simulink model "zumo_PID_controller_line_value"  (R2014b)
settings: Solver=ode3  SolverMode=SingleTasking  StartTime=0.0  StopTime=20  FixedStep=0.01  RelTol=1e-3
PreLoadFcn:
  | evalin('base','sim=1;');
InitFcn:
  | mapdata = processmap('mapTrackA.mat');
model workspace (MAT data in the model file):
  axleLength = Simulink.Parameter
  axleLength.Value = 9.8
  axleLength.Description = 'Distance between tire contact points
    | of the two wheels/treads
    | in units of centimeters.'
  axleLength.DataType = 'auto'
  commandPercmPerSecond = Simulink.Parameter
  commandPercmPerSecond.Value = 3.9547
  commandPercmPerSecond.Description = 'Convert units of ''command'' 
    | to units of ''cm/s''.
    | 
    | ''command'' is a value in the range [-256, 255].'
  commandPercmPerSecond.DataType = 'auto'
  symmetrizeMotors = Simulink.Parameter
  symmetrizeMotors.Value = 1
  symmetrizeMotors.Description = 'Scale one of the motor commands down 
    | (not up) to balance the motors. 
    | Once balanced, a value of x sent to either
    | motor will produce the same rate of rotation
    | in both motors.'
  symmetrizeMotors.DataType = 'auto'
  sampleTime = Simulink.Parameter
  sampleTime.Value = 0.01
  sampleTime.Description = 'Sample time (in seconds) of the trajectory simulator.'
  sampleTime.DataType = 'auto'
  commandThreshold = Simulink.Parameter
  commandThreshold.Value = 31.875
  commandThreshold.DataType = 'auto'
  lineThreshold = Simulink.Parameter
  lineThreshold.Value = 500
  lineThreshold.DataType = 'auto'
  velocity = Simulink.Parameter
  velocity.Value = 10
  velocity.Description = 'cm / s'
  velocity.DataType = 'auto'
  waveLength = Simulink.Parameter
  waveLength.Value = 8.6
  waveLength.Description = 'Units of cm.
    | 
    | The following condition must be satisfied: 
    | waveLength > 2*pi * velocity / sqrt(0.5 / sampleTime)
    | 
    | For reference,
    | robotLength = 8.6 cm
    | '
  waveLength.DataType = 'auto'
libraries: ZumoBotLib x2, simulink x1, arduinolib x1
settings Model: ExtModeTrigDuration=2  Creator=pkasseba  LastModifiedBy=sandip
settings OptimizationCC: OptimizeModelRefInitCode=on  LifeSpan=1
settings DebuggingCC: UnderspecifiedInitializationDetection=Classic  MergeDetectMultiDrivingBlocksExec=none  SolverPrmCheckMsg=none  StateNameClashWarn=warning
settings HardwareCC: ProdBitPerInt=16  ProdBitPerPointer=8  ProdIntDivRoundTo=Zero  ProdEndianess=LittleEndian  ProdWordSize=8  ProdHWDeviceType=Atmel->AVR
settings SFSimCC: SimParseCustomCode=off
settings RTWCC: SystemTargetFile=realtime.tlc  GenerateMakefile=off  TemplateMakefile=realtime.tmf  Description=Run on Target Hardware  RTWVerbose=off  ProcessScript=realtime_make_rtw_hook
settings STFCustomTargetCC: TargetLibSuffix=.a  GenerateSampleERTMain=on  ERTCustomFileBanners=on  SupportNonInlinedSFcns=off  SupportVariableSizeSignals=on  MATLABClassNameForMDSCustomization=Simulink.SoftwareTarget.ERTCustomization  GRTInterface=off  SystemTargetFile=realtime.tlc
settings ERTTargetCC: GenerateSampleERTMain=on  ParMdlRefBuildCompliant=off  CompOptLevelCompliant=off  ConcurrentExecutionCompliant=off  CombineOutputUpdateFcns=off  ERTFirstTimeCompliant=off  SupportContinuousTime=on  SupportVariableSizeSignals=on  ModelStepFunctionPrototypeControlCompliant=off  CPPClassGenCompliant=off  ExtModeTransport=3  ExtModeMexFile=ext_serial_win32_comm  ExtModeMexArgs=0 1 9600  InlinedParameterPlacement=NonHierarchical  ERTSrcFileBannerTemplate=realtime_code_template.cgt  ERTHdrFileBannerTemplate=realtime_code_template.cgt  ERTDataSrcFileTemplate=realtime_code_template.cgt  ERTDataHdrFileTemplate=realtime_code_template.cgt  ERTCustomFileTemplate=realtime_file_process.tlc

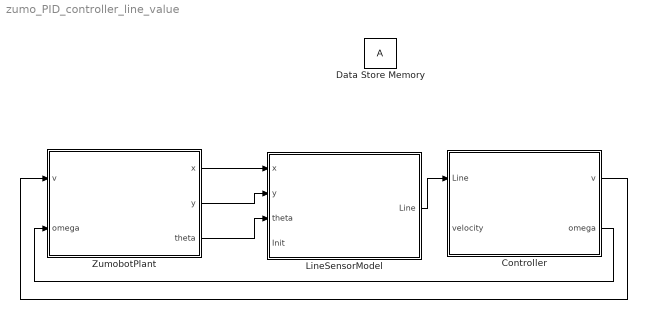
== system zumo_PID_controller_line_value ==
  Controller : Subsystem
  Data Store Memory : DataStoreMemory  Priority=2  ReadBeforeWriteMsg=warning  WriteAfterWriteMsg=warning  WriteAfterReadMsg=warning
  LineSensorModel : Subsystem  Variant=on
  ZumobotPlant : Subsystem  Variant=on
  wires:
  Controller/1(v) -> ZumobotPlant/1(v)
  ZumobotPlant/2(y) -> LineSensorModel/2(y)
  LineSensorModel/1(Line) -> Controller/1(Line)
  Controller/2(omega) -> ZumobotPlant/2(omega)
  ZumobotPlant/3(theta) -> LineSensorModel/3(theta)
  ZumobotPlant/1(x) -> LineSensorModel/1(x)

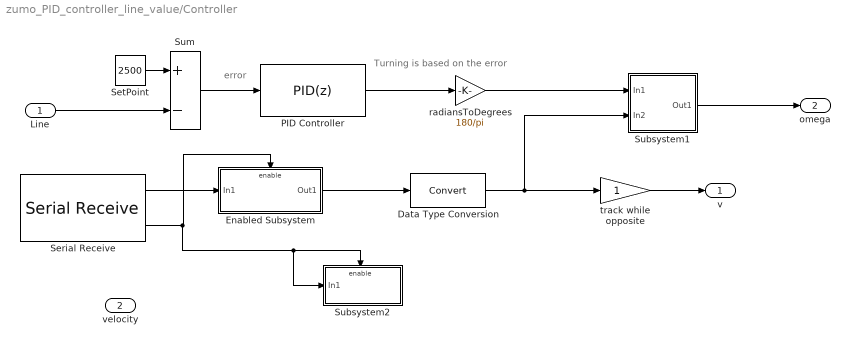
== system zumo_PID_controller_line_value/Controller ==
  note: Turning is based on the error
  note: error
  Line : Inport
  velocity : Inport  Port=2
  Data Type Conversion : DataTypeConversion
  Enabled Subsystem : Subsystem  TreatAsAtomicUnit=on
  PID Controller : simulink/Continuous/PID Controller  Controller=PID  TimeDomain=Discrete-time  SampleTime=-1  IntegratorMethod=Forward Euler  FilterMethod=Forward Euler  Form=Parallel  P=0.01  I=0.01  D=0.005  N=1  InitialConditionSource=internal  InitialConditionForIntegrator=0  InitialConditionForFilter=0  ExternalReset=none  LimitOutput=off  UpperSaturationLimit=5  LowerSaturationLimit=-5  LinearizeAsGain=on  AntiWindupMode=none  Kb=1  TrackingMode=off  Kt=1  PParamMin=[]  PParamMax=[]  IParamMin=[]  IParamMax=[]  DParamMin=[]  DParamMax=[]  NParamMin=[]  NParamMax=[]  KbParamMin=[]  KbParamMax=[]  KtParamMin=[]  KtParamMax=[]  POutMin=[]  POutMax=[]  IOutMin=[]  IOutMax=[]  DOutMin=[]  DOutMax=[]  NOutMin=[]  NOutMax=[]  KbOutMin=[]  KbOutMax=[]  KtOutMin=[]  KtOutMax=[]  IntegratorOutMin=[]  IntegratorOutMax=[]  FilterOutMin=[]  FilterOutMax=[]  SumOutMin=[]  SumOutMax=[]  SumI1OutMin=[]  SumI1OutMax=[]  SumI2OutMin=[]  SumI2OutMax=[]  SumI3OutMin=[]  SumI3OutMax=[]  SumDOutMin=[]  SumDOutMax=[]  SaturationOutMin=[]  SaturationOutMax=[]  IntegratorContinuousStateAttributes=''  IntegratorStateMustResolveToSignalObject=off  IntegratorRTWStateStorageClass=Auto  FilterContinuousStateAttributes=''  FilterStateMustResolveToSignalObject=off  FilterRTWStateStorageClass=Auto  DifferentiatorICPrevScaledInput=0  DifferentiatorOutMin=[]  DifferentiatorOutMax=[]  UseFilter=on
  Serial Receive : arduinolib/Serial Receive  portNumber=0  showOutStatus=on  sampleTime=0.01  blockPlatform=arduino
  SetPoint : Constant  Value=2500
  Subsystem1 : Subsystem
  Subsystem2 : Subsystem  Priority=0
  Sum : Sum  Inputs=+-
  radiansToDegrees : Gain  Gain=180/pi
  track while opposite : Gain
  v : Outport
  omega : Outport  Port=2
  wires:
  SetPoint/1 -> Sum/1
  Sum/1 -> PID Controller/1
  PID Controller/1 -> radiansToDegrees/1
  Line/1 -> Sum/2
  Data Type Conversion/1 -> Subsystem1/2(In2), track while opposite/1
  track while opposite/1 -> v/1
  radiansToDegrees/1 -> Subsystem1/1(In1)
  Subsystem1/1(Out1) -> omega/1
  Serial Receive/1 -> Enabled Subsystem/1(In1)
  Enabled Subsystem/1(Out1) -> Data Type Conversion/1
  Serial Receive/2 -> Subsystem2/1(In1), Subsystem2/Enable, Enabled Subsystem/Enable

== system zumo_PID_controller_line_value/LineSensorModel ==
  note: 1) Only subsystems can be added as variant choices at this level
      | 2) Blocks cannot be connected at this level as connectivity is
      | automatically determined at simulation, based on the active variant
  x : Inport
  y : Inport  Port=2
  theta : Inport  Port=3
  Init : Inport  Port=4
  Simulation : Subsystem  VariantControl=sim==1
  Target : Subsystem  VariantControl=sim==0
  Line : Outport

== system zumo_PID_controller_line_value/ZumobotPlant ==
  note: 1) Only subsystems can be added as variant choices at this level
      | 2) Blocks cannot be connected at this level as connectivity is
      | automatically determined at simulation, based on the active variant
  v : Inport
  omega : Inport  Port=2
  Simulation : Subsystem  VariantControl=sim==1
  Target : Subsystem  VariantControl=sim==0
  x : Outport
  y : Outport  Port=2
  theta : Outport  Port=3

== system zumo_PID_controller_line_value/Controller/Enabled Subsystem ==
  In1 : Inport
  Enable : EnablePort
  Out1 : Outport  InitialOutput=0
  wires:
  In1/1 -> Out1/1

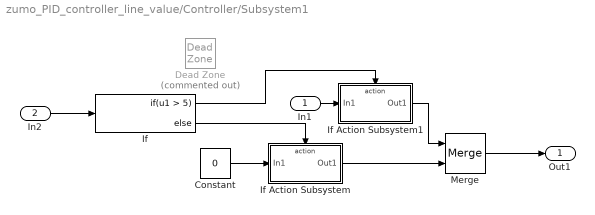
== system zumo_PID_controller_line_value/Controller/Subsystem1 ==
  In1 : Inport
  In2 : Inport  Port=2
  Constant : Constant  Value=0
  Dead Zone : DeadZone  Commented=on  LowerValue=-5  UpperValue=5  SaturateOnIntegerOverflow=on
  If : If  IfExpression=u1 > 5
  If Action Subsystem : Subsystem  TreatAsAtomicUnit=on
  If Action Subsystem1 : Subsystem  TreatAsAtomicUnit=on
  Merge : Merge
  Out1 : Outport
  wires:
  If/2 -> If Action Subsystem/Action
  Merge/1 -> Out1/1
  In2/1 -> If/1
  If Action Subsystem/1(Out1) -> Merge/2
  If Action Subsystem1/1(Out1) -> Merge/1
  In1/1 -> If Action Subsystem1/1(In1)
  Constant/1 -> If Action Subsystem/1(In1)
  If/1 -> If Action Subsystem1/Action

== system zumo_PID_controller_line_value/Controller/Subsystem2 ==
  In1 : Inport
  Enable : EnablePort
  Data Store Write : DataStoreWrite  DataStoreElements=A
  wires:
  In1/1 -> Data Store Write/1

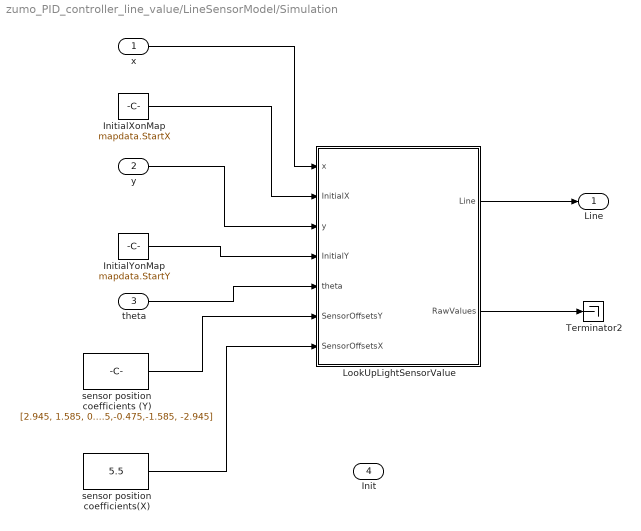
== system zumo_PID_controller_line_value/LineSensorModel/Simulation ==
  x : Inport
  y : Inport  Port=2
  theta : Inport  Port=3
  Init : Inport  Port=4
  InitialXonMap : Constant  Value=mapdata.StartX
  InitialYonMap : Constant  Value=mapdata.StartY
  LookUpLightSensorValue : Subsystem
  Terminator2 : Terminator
  sensor position coefficients (Y) : Constant  Value=[2.945, 1.585, 0.475,-0.475,-1.585, -2.945]
  sensor position coefficients(X) : Constant  Value=5.5
  Line : Outport
  wires:
  InitialYonMap/1 -> LookUpLightSensorValue/4(InitialY)
  theta/1 -> LookUpLightSensorValue/5(theta)
  sensor position coefficients (Y)/1 -> LookUpLightSensorValue/6(SensorOffsetsY)
  y/1 -> LookUpLightSensorValue/3(y)
  InitialXonMap/1 -> LookUpLightSensorValue/2(InitialX)
  x/1 -> LookUpLightSensorValue/1(x)
  sensor position coefficients(X)/1 -> LookUpLightSensorValue/7(SensorOffsetsX)
  LookUpLightSensorValue/1(Line) -> Line/1
  LookUpLightSensorValue/2(RawValues) -> Terminator2/1

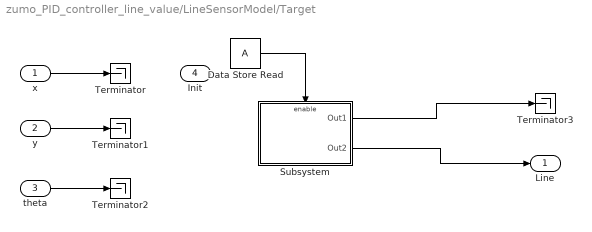
== system zumo_PID_controller_line_value/LineSensorModel/Target ==
  x : Inport
  y : Inport  Port=2
  theta : Inport  Port=3
  Init : Inport  Port=4
  Data Store Read : DataStoreRead
  Subsystem : Subsystem
  Terminator{,1..3} (4 alike) : Terminator
  Line : Outport
  wires:
  x/1 -> Terminator/1
  y/1 -> Terminator1/1
  theta/1 -> Terminator2/1
  Subsystem/1(Out1) -> Terminator3/1
  Subsystem/2(Out2) -> Line/1
  Data Store Read/1 -> Subsystem/Enable

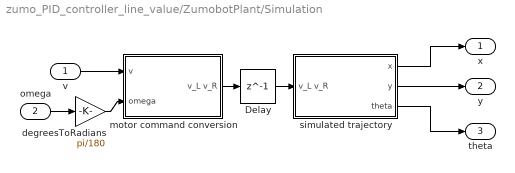
== system zumo_PID_controller_line_value/ZumobotPlant/Simulation ==
  v : Inport
  omega : Inport  Port=2
  Delay : Delay  DelayLength=1  InitialCondition=0
  degreesToRadians : Gain  Gain=pi/180
  motor command conversion : Subsystem
  simulated trajectory : Subsystem
  x : Outport
  y : Outport  Port=2
  theta : Outport  Port=3
  wires:
  v/1 -> motor command conversion/1(v)
  simulated trajectory/1(x) -> x/1
  simulated trajectory/2(y) -> y/1
  omega/1 -> degreesToRadians/1
  simulated trajectory/3(theta) -> theta/1
  degreesToRadians/1 -> motor command conversion/2(omega)
  motor command conversion/1(v_L v_R) -> Delay/1
  Delay/1 -> simulated trajectory/1(v_L v_R)

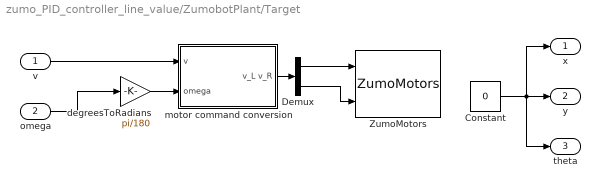
== system zumo_PID_controller_line_value/ZumobotPlant/Target ==
  v : Inport
  omega : Inport  Port=2
  Constant : Constant  Value=0
  Demux : Demux  Outputs=2
  ZumoMotors : ZumoBotLib/ZumoMotors  flipLeft=off  flipRight=off
  degreesToRadians : Gain  Gain=pi/180
  motor command conversion : Subsystem
  x : Outport
  y : Outport  Port=2
  theta : Outport  Port=3
  wires:
  motor command conversion/1(v_L v_R) -> Demux/1
  Demux/1 -> ZumoMotors/1
  Demux/2 -> ZumoMotors/2
  v/1 -> motor command conversion/1(v)
  omega/1 -> degreesToRadians/1
  Constant/1 -> theta/1, x/1, y/1
  degreesToRadians/1 -> motor command conversion/2(omega)

== system zumo_PID_controller_line_value/Controller/Subsystem1/If Action Subsystem ==
  In1 : Inport
  Action Port : ActionPort  ActionType=else
  Out1 : Outport
  wires:
  In1/1 -> Out1/1

== system zumo_PID_controller_line_value/Controller/Subsystem1/If Action Subsystem1 ==
  In1 : Inport
  Action Port : ActionPort  ActionType=then
  Out1 : Outport
  wires:
  In1/1 -> Out1/1

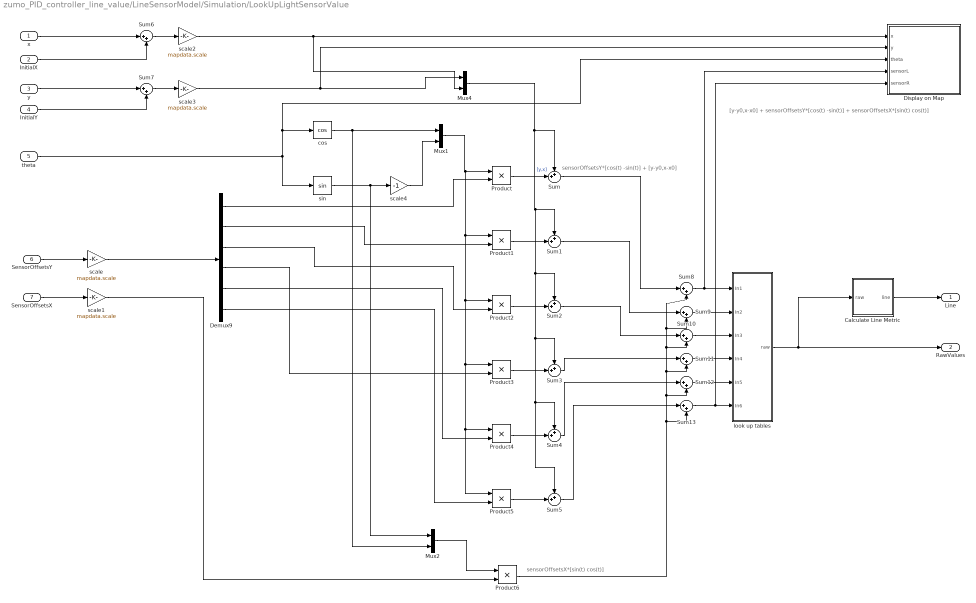
== system zumo_PID_controller_line_value/LineSensorModel/Simulation/LookUpLightSensorValue ==
  note: [y-y0,x-x0] + sensorOffsetsY*[cos(t) -sin(t)] + sensorOffsetsX*[sin(t) cos(t)]
  note: sensorOffsetsY*[cos(t) -sin(t)] + [y-y0,x-x0]
  note: sensorOffsetsX*[sin(t) cos(t)]
  x : Inport
  InitialX : Inport  Port=2
  y : Inport  Port=3
  InitialY : Inport  Port=4
  theta : Inport  Port=5
  SensorOffsetsY : Inport  Port=6
  SensorOffsetsX : Inport  Port=7
  Calculate Line Metric : Subsystem
  Demux9 : Demux  Outputs=6
  Display on Map : MATLAB Function  TreatAsAtomicUnit=on
  Mux1 : Mux  Inputs=2
  Mux2 : Mux  Inputs=2
  Mux4 : Mux  Inputs=2
  Product{,1..6} (7 alike) : Product
  Sum{,1..5} (6 alike) : Sum  Inputs=++|
  Sum{6..13} (8 alike) : Sum  Inputs=|++
  cos : Trigonometry  Operator=cos
  look up tables : Subsystem
  scale{,1..3} (4 alike) : Gain  Gain=mapdata.scale
  scale4 : Gain  Gain=-1
  sin : Trigonometry
  Line : Outport
  RawValues : Outport  Port=2
  wires:
  SensorOffsetsY/1 -> scale/1
  Mux1/1 -> Product5/1, Product4/1, Product3/1, Product2/1, Product1/1, Product/1
  Product/1 -> Sum/2
  Product1/1 -> Sum1/2
  Product2/1 -> Sum2/2
  Product4/1 -> Sum4/2
  Product3/1 -> Sum3/2
  Product5/1 -> Sum5/2
  Sum/1 -> Sum8/1
  Sum5/1 -> Sum13/1
  scale/1 -> Demux9/1
  Demux9/4 -> Product3/2
  Demux9/5 -> Product4/2
  Demux9/3 -> Product2/2
  Demux9/6 -> Product5/2
  Demux9/2 -> Product1/2
  Demux9/1 -> Product/2
  Mux4/1 -> Sum/1, Sum5/1, Sum4/1, Sum3/1, Sum2/1, Sum1/1  "[y,x]"
  SensorOffsetsX/1 -> scale1/1
  scale1/1 -> Product6/2
  Mux2/1 -> Product6/1
  Product6/1 -> Sum13/2, Sum12/2, Sum11/2, Sum10/2, Sum9/2, Sum8/2
  x/1 -> Sum6/1
  Sum6/1 -> scale2/1
  InitialX/1 -> Sum6/2
  y/1 -> Sum7/1
  Sum7/1 -> scale3/1
  InitialY/1 -> Sum7/2
  scale2/1 -> Mux4/2, Display on Map/1(x)
  scale3/1 -> Mux4/1, Display on Map/2(y)
  Calculate Line Metric/1(line) -> Line/1
  look up tables/1(raw) -> Calculate Line Metric/1(raw), RawValues/1
  Sum1/1 -> Sum9/1
  Sum2/1 -> Sum10/1
  Sum3/1 -> Sum11/1
  Sum4/1 -> Sum12/1
  Sum8/1 -> Display on Map/4(sensorL), look up tables/1(In1)
  Sum9/1 -> look up tables/2(In2)
  Sum10/1 -> look up tables/3(In3)
  Sum11/1 -> look up tables/4(In4)
  Sum12/1 -> look up tables/5(In5)
  Sum13/1 -> Display on Map/5(sensorR), look up tables/6(In6)
  sin/1 -> Mux2/1, scale4/1
  cos/1 -> Mux2/2, Mux1/1
  theta/1 -> Display on Map/3(theta), cos/1, sin/1
  scale4/1 -> Mux1/2

== system zumo_PID_controller_line_value/LineSensorModel/Target/Subsystem ==
  Enable : EnablePort
  ZumoReflectanceSensor : ZumoBotLib/ZumoReflectanceSensor  sampleTime_dd=0.01  emitterPin_dd=255  debug_dd=off
  Out1 : Outport
  Out2 : Outport  Port=2  InitialOutput=2500
  wires:
  ZumoReflectanceSensor/2 -> Out2/1
  ZumoReflectanceSensor/1 -> Out1/1

== system zumo_PID_controller_line_value/ZumobotPlant/Simulation/motor command conversion ==
  note: or in matrix notation,
  note: v_L  = v - omega * axleLength/2
      | v_R = v + omega * axleLength/2
  note: [v_L; v_R] = [1 -axleLength/2; 1 axleLength/2] * [v; omega]
  v : Inport
  omega : Inport  Port=2
  Mux : Mux  Inputs=2
  Saturation [-256 255] : Saturate  UpperLimit=255  LowerLimit=-256
  change parameters : Gain  Gain=[1 -axleLength/2; 1 axleLength/2]  Multiplication=Matrix(K*u)
  change units : Gain  Gain=commandPercmPerSecond
  symmetrize motors : Gain  Gain=[1 symmetrizeMotors]
  v_L v_R : Outport
  wires:
  change parameters/1 -> symmetrize motors/1  "v_L v_R"
  change units/1 -> Saturation [-256 255]/1  "v_L v_R (command)"
  symmetrize motors/1 -> change units/1  "v_L v_R (cm/s)"
  Saturation [-256 255]/1 -> v_L v_R/1
  Mux/1 -> change parameters/1
  omega/1 -> Mux/2
  v/1 -> Mux/1

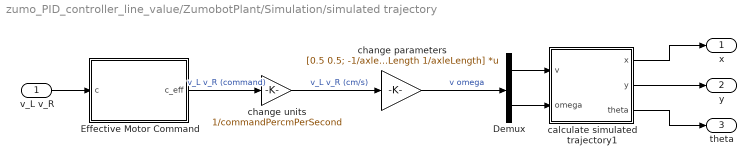
== system zumo_PID_controller_line_value/ZumobotPlant/Simulation/simulated trajectory ==
  v_L v_R : Inport
  Demux : Demux  Outputs=2
  Effective Motor Command : Subsystem
  calculate simulated trajectory1 : Subsystem
  change parameters : Gain  Gain=[0.5 0.5; -1/axleLength 1/axleLength]  Multiplication=Matrix(K*u)
  change units : Gain  Gain=1/commandPercmPerSecond
  x : Outport
  y : Outport  Port=2
  theta : Outport  Port=3
  wires:
  Demux/2 -> calculate simulated trajectory1/2(omega)
  Demux/1 -> calculate simulated trajectory1/1(v)
  v_L v_R/1 -> Effective Motor Command/1(c)
  Effective Motor Command/1(c_eff) -> change units/1  "v_L v_R (command)"
  change units/1 -> change parameters/1  "v_L v_R (cm/s)"
  change parameters/1 -> Demux/1  "v omega"
  calculate simulated trajectory1/2(y) -> y/1
  calculate simulated trajectory1/3(theta) -> theta/1
  calculate simulated trajectory1/1(x) -> x/1

== system zumo_PID_controller_line_value/ZumobotPlant/Target/motor command conversion ==
  note: or in matrix notation,
  note: v_L  = v - omega * axleLength/2
      | v_R = v + omega * axleLength/2
  note: [v_L; v_R] = [1 -axleLength/2; 1 axleLength/2] * [v; omega]
  v : Inport
  omega : Inport  Port=2
  Mux : Mux  Inputs=2
  Saturation [-256 255] : Saturate  UpperLimit=255  LowerLimit=-256
  change parameters : Gain  Gain=[1 -axleLength/2; 1 axleLength/2]  Multiplication=Matrix(K*u)
  change units : Gain  Gain=commandPercmPerSecond
  symmetrize motors : Gain  Gain=[1 symmetrizeMotors]
  v_L v_R : Outport
  wires:
  change parameters/1 -> symmetrize motors/1  "v_L v_R"
  change units/1 -> Saturation [-256 255]/1  "v_L v_R (command)"
  symmetrize motors/1 -> change units/1  "v_L v_R (cm/s)"
  Saturation [-256 255]/1 -> v_L v_R/1
  Mux/1 -> change parameters/1
  omega/1 -> Mux/2
  v/1 -> Mux/1

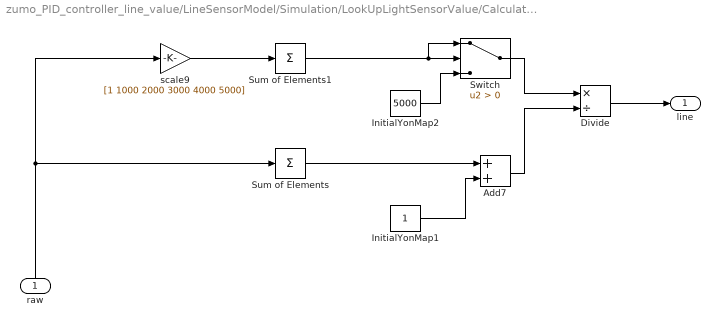
== system zumo_PID_controller_line_value/LineSensorModel/Simulation/LookUpLightSensorValue/Calculate Line Metric ==
  raw : Inport
  Add7 : Sum
  Divide : Product  Inputs=*/
  InitialYonMap1 : Constant
  InitialYonMap2 : Constant  Value=5000
  Sum of Elements : Sum  Inputs=+
  Sum of Elements1 : Sum  Inputs=+
  Switch : Switch  Criteria=u2 > Threshold
  scale9 : Gain  Gain=[1 1000 2000 3000 4000 5000]
  line : Outport
  wires:
  Sum of Elements/1 -> Add7/1
  Divide/1 -> line/1
  InitialYonMap1/1 -> Add7/2
  Add7/1 -> Divide/2
  Sum of Elements1/1 -> Switch/1, Switch/2
  Switch/1 -> Divide/1
  InitialYonMap2/1 -> Switch/3
  scale9/1 -> Sum of Elements1/1
  raw/1 -> scale9/1, Sum of Elements/1

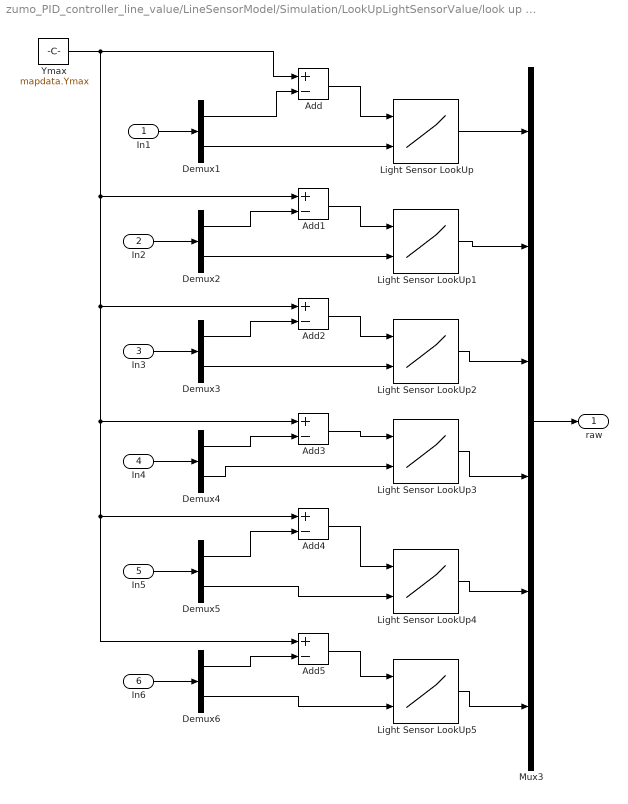
== system zumo_PID_controller_line_value/LineSensorModel/Simulation/LookUpLightSensorValue/look up tables ==
  In1 : Inport
  In2 : Inport  Port=2
  In3 : Inport  Port=3
  In4 : Inport  Port=4
  In5 : Inport  Port=5
  In6 : Inport  Port=6
  Add{,1..5} (6 alike) : Sum  Inputs=+-
  Demux{1..6} (6 alike) : Demux  Outputs=2
  Light Sensor LookUp{,1..5} (6 alike) : Lookup_n-D  BreakpointsForDimension1=mapdata.yBreakPoints  BreakpointsForDimension2=mapdata.xBreakPoints  Table=mapdata.ReflectanceData  InterpMethod=Flat  ExtrapMethod=Clip  UseLastTableValue=on  RndMeth=Round  SaturateOnIntegerOverflow=on  InputSameDT=on
  Mux3 : Mux  Inputs=6
  Ymax : Constant  Value=mapdata.Ymax
  raw : Outport
  wires:
  Demux1/1 -> Add/2
  Demux1/2 -> Light Sensor LookUp/2
  Demux2/2 -> Light Sensor LookUp1/2
  In2/1 -> Demux2/1
  Demux3/2 -> Light Sensor LookUp2/2
  Demux4/2 -> Light Sensor LookUp3/2
  Demux5/2 -> Light Sensor LookUp4/2
  Demux6/2 -> Light Sensor LookUp5/2
  In3/1 -> Demux3/1
  In4/1 -> Demux4/1
  In5/1 -> Demux5/1
  Light Sensor LookUp4/1 -> Mux3/5
  Light Sensor LookUp1/1 -> Mux3/2
  Light Sensor LookUp5/1 -> Mux3/6
  Light Sensor LookUp3/1 -> Mux3/4
  Light Sensor LookUp2/1 -> Mux3/3
  Light Sensor LookUp/1 -> Mux3/1
  Mux3/1 -> raw/1
  Add/1 -> Light Sensor LookUp/1
  Demux2/1 -> Add1/2
  Add1/1 -> Light Sensor LookUp1/1
  Demux3/1 -> Add2/2
  Add2/1 -> Light Sensor LookUp2/1
  Demux4/1 -> Add3/2
  Add3/1 -> Light Sensor LookUp3/1
  Demux5/1 -> Add4/2
  Add4/1 -> Light Sensor LookUp4/1
  Demux6/1 -> Add5/2
  Ymax/1 -> Add5/1, Add4/1, Add3/1, Add2/1, Add1/1, Add/1
  Add5/1 -> Light Sensor LookUp5/1
  In6/1 -> Demux6/1
  In1/1 -> Demux1/1

== system zumo_PID_controller_line_value/ZumobotPlant/Simulation/simulated trajectory/Effective Motor Command ==
  note: Zumobot does not move when given a command
      | with an abs less than 50 on a smooth surface,
      | so such commands are effectively 0.
  note: Do not saturate this signal.The process of symmetrizing
      | the motor commands gives rise to this artificial signal,
      | which can exceed the value of 255.
  c : Inport
  Abs : Abs
  Constant1 : Constant  Value=0
  Sum : Sum  Inputs=|+-
  Switch : Switch
  command threshold : Constant  Value=commandThreshold
  symmetrize motors : Gain  Gain=[1 1/symmetrizeMotors]
  c_eff : Outport
  wires:
  Switch/1 -> c_eff/1
  symmetrize motors/1 -> Abs/1, Switch/1
  Sum/1 -> Switch/2
  Abs/1 -> Sum/1
  command threshold/1 -> Sum/2
  c/1 -> symmetrize motors/1  "v_L v_R"
  Constant1/1 -> Switch/3

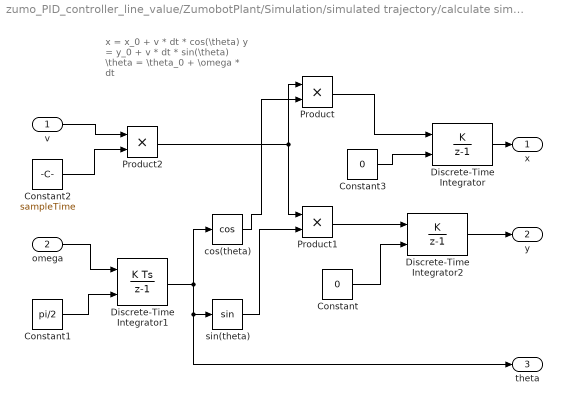
== system zumo_PID_controller_line_value/ZumobotPlant/Simulation/simulated trajectory/calculate simulated trajectory1 ==
  note: x = x_0 + v * dt * cos(\theta)
      | y = y_0 + v * dt * sin(\theta)
      | \theta = \theta_0 + \omega * dt
  v : Inport
  omega : Inport  Port=2
  Constant : Constant  Value=0
  Constant1 : Constant  Value=pi/2
  Constant2 : Constant  Value=sampleTime
  Constant3 : Constant  Value=0
  Discrete-Time Integrator : DiscreteIntegrator  IntegratorMethod=Accumulation: Forward Euler  InitialConditionSource=external  InitialConditionSetting=State (most efficient)  SampleTime=-1
  Discrete-Time Integrator1 : DiscreteIntegrator  InitialConditionSource=external  SampleTime=-1
  Discrete-Time Integrator2 : DiscreteIntegrator  IntegratorMethod=Accumulation: Forward Euler  InitialConditionSource=external  InitialConditionSetting=State (most efficient)  SampleTime=-1
  Product : Product
  Product1 : Product
  Product2 : Product
  cos(theta) : Trigonometry  Operator=cos
  sin(theta) : Trigonometry
  x : Outport
  y : Outport  Port=2
  theta : Outport  Port=3
  wires:
  omega/1 -> Discrete-Time Integrator1/1
  v/1 -> Product2/1
  Discrete-Time Integrator1/1 -> theta/1, sin(theta)/1, cos(theta)/1
  Product/1 -> Discrete-Time Integrator/1
  cos(theta)/1 -> Product/2
  Product2/1 -> Product/1, Product1/1
  sin(theta)/1 -> Product1/2
  Constant3/1 -> Discrete-Time Integrator/2
  Constant1/1 -> Discrete-Time Integrator1/2
  Constant2/1 -> Product2/2
  Discrete-Time Integrator/1 -> x/1
  Product1/1 -> Discrete-Time Integrator2/1
  Discrete-Time Integrator2/1 -> y/1
  Constant/1 -> Discrete-Time Integrator2/2

== matlab function zumo_PID_controller_line_value/LineSensorModel/Simulation/LookUpLightSensorValue/Display on Map ==
  data: x input; y input; theta input; sensorL input; sensorR input
function fcn(x,y, theta, sensorL,sensorR)
%#codegen

coder.extrinsic('dispOnMap');
dispOnMap(x,y, theta, sensorL, sensorR);
